simulink model "slexEntityTransportDelay_fixed"  (R2022b)
settings: Solver=FixedStepAuto  StartTime=0.0  StopTime=timeFinal  FixedStep=timeStepMax  RelTol=1e-3
PostLoadFcn:
  | Simulink.defineIntEnumType('OperationMode', {'Idle', 'OnDemand', 'Max'}, [0; 1; 2]);
Description:
  | <include>VariableSpeedConveyorBeltExample.m</include>
settings Model: PacingRate=1000  Creator=The MathWorks, Inc.  LastModifiedBy=jun
settings SolverCC: AlgebraicLoopSolver=TrustRegion
settings DataIOCC: ExternalInput=ds  LoadExternalInput=on
settings DebuggingCC: UnconnectedInputMsg=warning  UnconnectedOutputMsg=warning  UnconnectedLineMsg=warning  StrictBusMsg=ErrorOnBusTreatedAsVector  SymbolicDimsDataTypeCodeGenerationDiagnostic=none  SFMachineParentedDataDiag=warning
settings ModelReferenceCC: EnableRefExpFcnMdlSchedulingChecks=on

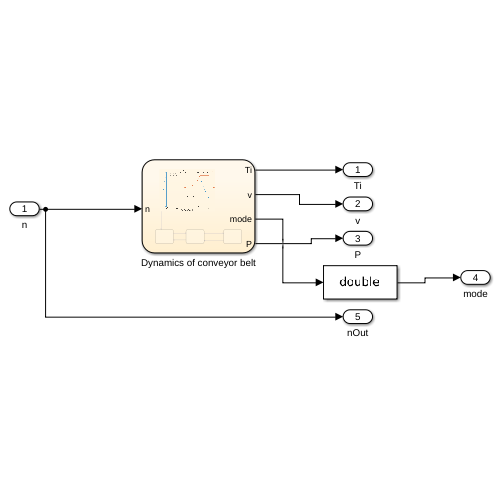
[thumbnail: Simulink's stored preview of the top-level diagram]
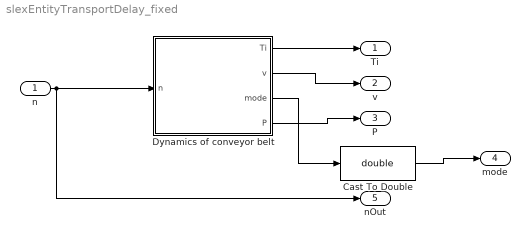
== system slexEntityTransportDelay_fixed ==
  n : Inport  OutDataTypeStr=double
  Cast To Double : DataTypeConversion  OutDataTypeStr=double  SaturateOnIntegerOverflow=off  RndMeth=Floor
  Dynamics of conveyor belt : Stateflow chart  TreatAsAtomicUnit=on
      settings: PortSchema="{\"entries\":[{\"content\":{\"sides\":[{\"content\":{\"connectorIds\":[\"In1\"]},\"type\":\"ConnectorPlacement.EquallySpacedRectSide\",\"uuid\":\"ddefda4b-8747-4a4a-a1d3-e21bd3366c18\"},{\"content\":{\"connectorIds\":[\"Out1\",\"Out2\",\"Out4\",\"Out3\"],\"side\":\"RIGHT\"},\"type\":\"ConnectorPlacement.EquallySpacedRectSide\",\"uuid\":\"5d88a7fa-e176-41b2-9696-d3f74e185f36\"},{\"content\":{\"connectorIds\":[],\"side\":\"TOP\"},\"type\":\"ConnectorPlacement.EquallySpacedRectSide\",\"uuid\":\"87e85ede-03e5-496a-9bed-db798efa9927\"}]},\"type\":\"ConnectorPlacement.EquallySpacedConnector\",\"uuid\":\"b01d8029-1168-4b3f-af55-c636f8f116eb\"}],\"packageUris\":[\"http://schema.mathworks.com/mf0/Connector/R2020b\"],\"version\":\"1.0\"}"
  Ti : Outport  OutDataTypeStr=double
  v : Outport  Port=2  OutDataTypeStr=double
  P : Outport  Port=3  OutDataTypeStr=double
  mode : Outport  Port=4  OutDataTypeStr=double
  nOut : Outport  Port=5
  wires:
  Dynamics of conveyor belt/1(Ti) -> Ti/1
  Dynamics of conveyor belt/2(v) -> v/1
  Dynamics of conveyor belt/3(P) -> P/1
  n/1 -> nOut/1, Dynamics of conveyor belt/1(n)
  Cast To Double/1 -> mode/1
  Dynamics of conveyor belt/4(mode) -> Cast To Double/1

== stateflow chart slexEntityTransportDelay_fixed/Dynamics of conveyor belt ==
  note: ?
  state Idle
    % no load
    Ti=100;
    v=1/Ti*L;
    P=(mu*n+fBelt)*v;
    mode=0;
  state OnDemand
    % keep speed
    Ti=L/V;
    v=V;
    P=(mu*n+fBelt)*v;
    mode=1;
  state Max
    % keep power
    v=maxPower/(mu*n+fBelt);
    Ti = L/v;
    P=(mu*n+fBelt)*v;
    mode=2;
  (default) -> Idle : {
      | % initialize local parameters
      | aveMass = 75;
      | mu = 0.5*10*aveMass; % *mu*g*aveMass, [N]
      | maxPower = 5e4; % maximum power, [W]
      | V = 3; % normal mode velocity, [m/s]
      | L = 50; % length of belt, [L]
      | fBelt = 1e4; % friction of zero load, [N]
      | }
  Idle -> OnDemand : [n*aveMass >= 10]
  OnDemand -> Max [order 2] : [(maxPower/V-fBelt)/mu  <= n]
  OnDemand -> Idle [order 1] : [n*aveMass < 10]
  Max -> OnDemand : [(maxPower/V-fBelt)/mu > n]
  data: Ti output; n input; mu local double =50; maxPower local double =5e4; V local double =3; L local double =50; fBelt local double =1e4; v output; P output; mode output int8; aveMass local
